simulink model "master_mult"  (R2015a)
settings: Solver=ode45  StartTime=0.0  StopTime=10.0  RelTol=1e-3
undefined symbols (not defined in the file): NumBits1, NumBits2, Slope1, Slope2
libraries: simulink x4
settings Model: Creator=acook  LastModifiedBy=ACook
settings DataIOCC: LimitDataPoints=off
settings HardwareCC: ProdHWDeviceType=ASIC/FPGA  TargetHWDeviceType=Generic->Unspecified (assume 32-bit Generic)  ProdEqTarget=off

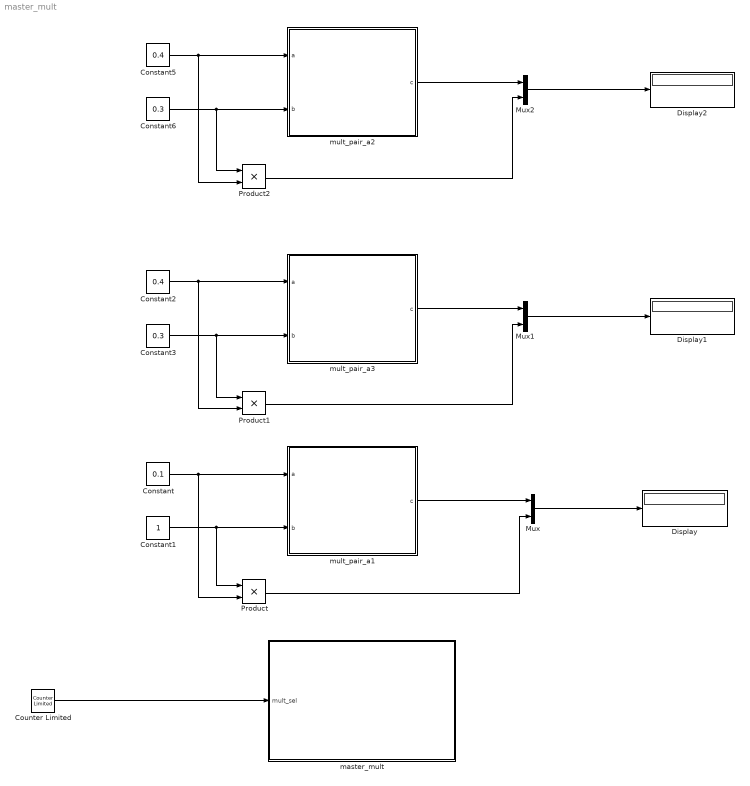
== system master_mult ==
  Constant : Constant  Value=0.1  OutDataTypeStr=fixdt(1,9,9)  SampleTime=-1
  Constant1 : Constant  OutDataTypeStr=fixdt(0,10,10)
  Constant2 : Constant  Value=0.4  OutDataTypeStr=fixdt(1,10,10)
  Constant3 : Constant  Value=0.3  OutDataTypeStr=fixdt(1,6,6)
  Constant5 : Constant  Value=0.4  OutDataTypeStr=fixdt(0,10,10)
  Constant6 : Constant  Value=0.3  OutDataTypeStr=fixdt(0,6,6)
  Counter Limited : simulink/Sources/Counter Limited  uplimit=7  tsamp=1
  Display : Display
  Display1 : Display
  Display2 : Display
  Mux : Mux  Inputs=2
  Mux1 : Mux  Inputs=2
  Mux2 : Mux  Inputs=2
  Product : Product
  Product1 : Product
  Product2 : Product
  master_mult : Subsystem
  mult_pair_a1 : Subsystem  mask{mult_tag=a}
      mask prompts: mult_tag "Mult Pair Prefix"
      mask Callback mult_tag:
      | tag = get_param(gcb,'mult_tag');
      | 
      | b = find_system(gcb,'LookUnderMasks','all','BlockType','Goto');
      | set_param(b{1},'GotoTag', [tag , '_master_mult_in']);
      mask Display: image('multiply_img.png',[.2 .2 .6 .6])
  mult_pair_a2 : Subsystem  mask{mult_tag=c}
      mask prompts: mult_tag "Mult Pair Prefix"
      mask Callback mult_tag:
      | tag = get_param(gcb,'mult_tag');
      | 
      | b = find_system(gcb,'LookUnderMasks','all','BlockType','Goto');
      | set_param(b{1},'GotoTag', [tag , '_master_mult_in']);
      mask Display: image('multiply_img.png',[.2 .2 .6 .6])
  mult_pair_a3 : Subsystem  mask{mult_tag=b}
      mask prompts: mult_tag "Mult Pair Prefix"
      mask Callback mult_tag:
      | tag = get_param(gcb,'mult_tag');
      | 
      | b = find_system(gcb,'LookUnderMasks','all','BlockType','Goto');
      | set_param(b{1},'GotoTag', [tag , '_master_mult_in']);
      mask Display: image('multiply_img.png',[.2 .2 .6 .6])
  wires:
  Constant/1 -> mult_pair_a1/1(a), Product/2
  Constant1/1 -> mult_pair_a1/2(b), Product/1
  mult_pair_a1/1(c) -> Mux/1
  Counter Limited/1 -> master_mult/1(mult_sel)
  Product/1 -> Mux/2
  Mux/1 -> Display/1
  mult_pair_a3/1(c) -> Mux1/1
  Constant2/1 -> mult_pair_a3/1(a), Product1/2
  Constant3/1 -> mult_pair_a3/2(b), Product1/1
  Product1/1 -> Mux1/2
  Mux1/1 -> Display1/1
  mult_pair_a2/1(c) -> Mux2/1
  Constant5/1 -> mult_pair_a2/1(a), Product2/2
  Constant6/1 -> mult_pair_a2/2(b), Product2/1
  Product2/1 -> Mux2/2
  Mux2/1 -> Display2/1

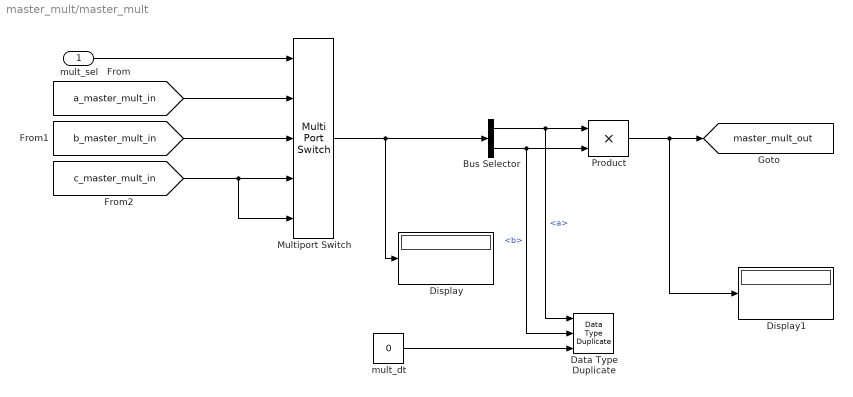
== system master_mult/master_mult ==
  mult_sel : Inport
  Bus Selector : BusSelector  OutputSignals=a,b
  Data Type Duplicate : DataTypeDuplicate  NumInputPorts=3
  Display : Display
  Display1 : Display
  Multiport Switch : MultiPortSwitch  DataPortOrder=Zero-based contiguous  Inputs=4
  Product : Product
  mult_dt : Constant  Value=0  OutDataTypeStr=SP.MULT_DT  SampleTime=-1
  tag scope: master_mult_out=global
  wires:
  mult_sel/1 -> Multiport Switch/1
  Multiport Switch/1 -> Display/1, Bus Selector/1
  Bus Selector/1 -> Data Type Duplicate/1, Product/1  "<a>"
  Bus Selector/2 -> Data Type Duplicate/2, Product/2  "<b>"
  Product/1 -> Display1/1, [master_mult_out]
  mult_dt/1 -> Data Type Duplicate/3
  [a_master_mult_in] -> Multiport Switch/2
  [b_master_mult_in] -> Multiport Switch/3
  [c_master_mult_in] -> Multiport Switch/5, Multiport Switch/4

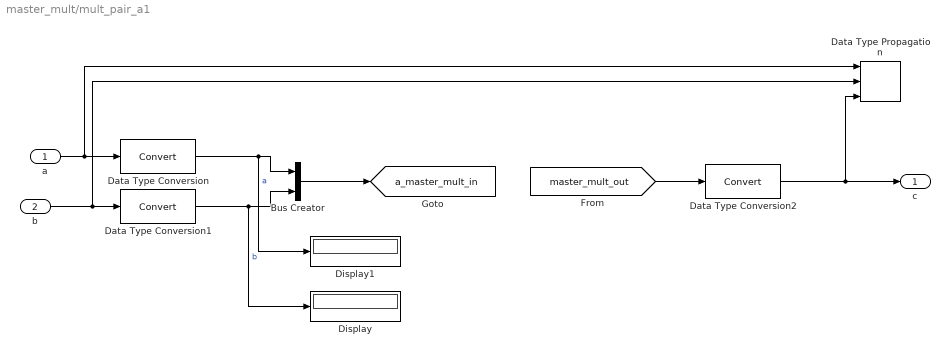
== system master_mult/mult_pair_a1 ==
  a : Inport
  b : Inport  Port=2
  Bus Creator : BusCreator  Inputs=2
  Data Type Propagation : simulink/Signal Attributes/Data Type Propagation  PropDataType=fixdt(1, 16)  IfRefDouble=double  IfRefSingle=single  IsSigned=IsSigned1 or IsSigned2  NumBitsBase=NumBits1+NumBits2  NumBitsMult=1  NumBitsAdd=0  NumBitsAllowFinal=1:128  PropScaling=2^-10  ValuesUsedBestPrec=[5 -7]  SlopeBase=Slope1*Slope2  SlopeMult=1  SlopeAdd=0  BiasBase=Bias1  BiasMult=1  BiasAdd=0
  Data Type Conversion : DataTypeConversion
  Data Type Conversion1 : DataTypeConversion
  Data Type Conversion2 : DataTypeConversion
  Display : Display
  Display1 : Display
  c : Outport
  tag scope: a_master_mult_in=global
  wires:
  Bus Creator/1 -> [a_master_mult_in]
  [master_mult_out] -> Data Type Conversion2/1
  b/1 -> Data Type Propagation/2, Data Type Conversion1/1
  a/1 -> Data Type Propagation/1, Data Type Conversion/1
  Data Type Conversion/1 -> Bus Creator/1, Display1/1  "a"
  Data Type Conversion1/1 -> Bus Creator/2, Display/1  "b"
  Data Type Conversion2/1 -> Data Type Propagation/3, c/1

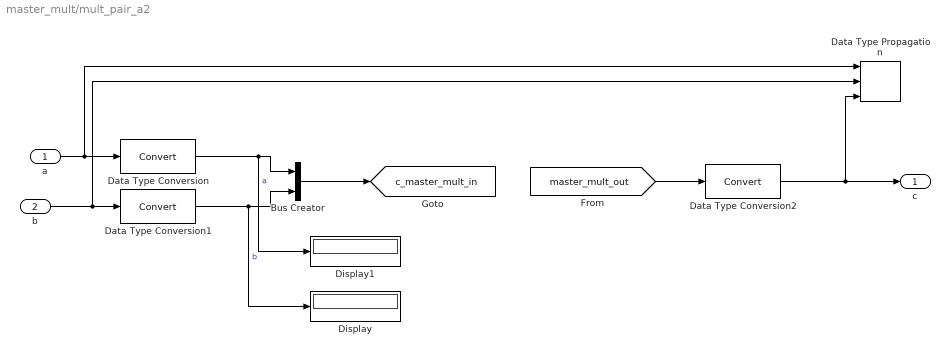
== system master_mult/mult_pair_a2 ==
  a : Inport
  b : Inport  Port=2
  Bus Creator : BusCreator  Inputs=2
  Data Type Propagation : simulink/Signal Attributes/Data Type Propagation  PropDataType=fixdt(1, 16)  IfRefDouble=double  IfRefSingle=single  IsSigned=IsSigned1 or IsSigned2  NumBitsBase=NumBits1+NumBits2  NumBitsMult=1  NumBitsAdd=0  NumBitsAllowFinal=1:128  PropScaling=2^-10  ValuesUsedBestPrec=[5 -7]  SlopeBase=Slope1*Slope2  SlopeMult=1  SlopeAdd=0  BiasBase=Bias1  BiasMult=1  BiasAdd=0
  Data Type Conversion : DataTypeConversion
  Data Type Conversion1 : DataTypeConversion
  Data Type Conversion2 : DataTypeConversion
  Display : Display
  Display1 : Display
  c : Outport
  tag scope: c_master_mult_in=global
  wires:
  Bus Creator/1 -> [c_master_mult_in]
  [master_mult_out] -> Data Type Conversion2/1
  b/1 -> Data Type Propagation/2, Data Type Conversion1/1
  a/1 -> Data Type Propagation/1, Data Type Conversion/1
  Data Type Conversion/1 -> Bus Creator/1, Display1/1  "a"
  Data Type Conversion1/1 -> Bus Creator/2, Display/1  "b"
  Data Type Conversion2/1 -> Data Type Propagation/3, c/1

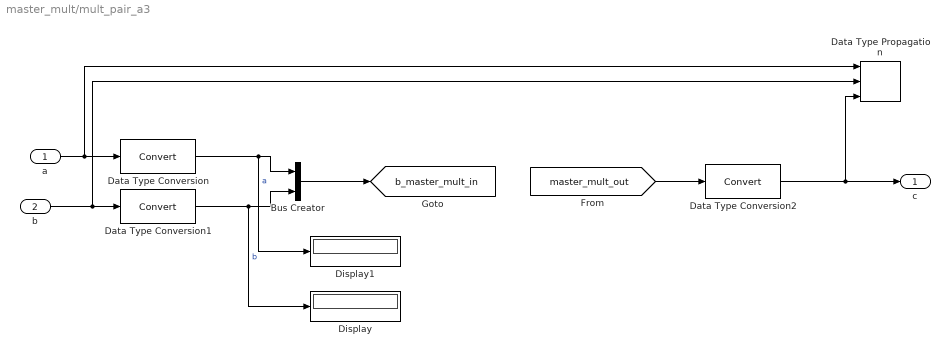
== system master_mult/mult_pair_a3 ==
  a : Inport
  b : Inport  Port=2
  Bus Creator : BusCreator  Inputs=2
  Data Type Propagation : simulink/Signal Attributes/Data Type Propagation  PropDataType=fixdt(1, 16)  IfRefDouble=double  IfRefSingle=single  IsSigned=IsSigned1 or IsSigned2  NumBitsBase=NumBits1+NumBits2  NumBitsMult=1  NumBitsAdd=0  NumBitsAllowFinal=1:128  PropScaling=2^-10  ValuesUsedBestPrec=[5 -7]  SlopeBase=Slope1*Slope2  SlopeMult=1  SlopeAdd=0  BiasBase=Bias1  BiasMult=1  BiasAdd=0
  Data Type Conversion : DataTypeConversion
  Data Type Conversion1 : DataTypeConversion
  Data Type Conversion2 : DataTypeConversion
  Display : Display
  Display1 : Display
  c : Outport
  tag scope: b_master_mult_in=global
  wires:
  Bus Creator/1 -> [b_master_mult_in]
  [master_mult_out] -> Data Type Conversion2/1
  b/1 -> Data Type Propagation/2, Data Type Conversion1/1
  a/1 -> Data Type Propagation/1, Data Type Conversion/1
  Data Type Conversion/1 -> Bus Creator/1, Display1/1  "a"
  Data Type Conversion1/1 -> Bus Creator/2, Display/1  "b"
  Data Type Conversion2/1 -> Data Type Propagation/3, c/1
